simulink model "Main_bikesim_ontest2"  (R2024b)
settings: Solver=FixedStepAuto  StartTime=0.0  StopTime=inf  FixedStep=0.0005
values from neighbouring files (symbols this model uses):
  A_d = permute(A_d,[1,3,2])    [Main_sim.m]    (also in Startup_labview_v2.m; sensor_error_test_sequence.m = (eye(size(A))+Ts*A))
  Ad_t = eye(1)+Ts*A_t    [Main_sim.m]    (also in Startup_labview_v2.m = (eye(size(A_t))+Ts*A_t))
  B_d = zeros(V_n,7,1)    [Main_sim.m]    (also in Startup_labview_v2.m; sensor_error_test_sequence.m = Ts*B)
  badGPS = 0    [Main_sim.m]
  Bd_t = B_t*Ts    [Main_sim.m]    (also in Startup_labview_v2.m)
  bike_model = 1    [Main_sim.m]
  bike_params = LoadBikeParameters(bike)    [Compare_real_to_sim.m]    (also in MPC_Data_train.m = LoadBikeParameters("green"); Main_sim.m; Startup_labview_v2.m; sensor_error_test_sequence.m)
  C = mpc_outer_params.Cd    [MPC_Data_train.m]    (also in Main_sim.m = permute(C,[1,3,2]); Startup_labview_v2.m = permute(C,[1,3,2]); fromIMU2trajectory.m = (W_roll * W_roll.') / max(1, size(W_roll,2)); sensor_data_check.m = (W_roll * W_roll.') / max(1, size(W_roll,2)))
  C_t = zeros(V_n,1)    [Main_sim.m]    (also in Startup_labview_v2.m)
  counter = zeros(V_n,1)    [Main_sim.m]    (also in Startup_labview_v2.m; sensor_error_test_sequence.m = 9)
  D = mpc_outer_params.Dd    [MPC_Data_train.m]    (also in Main_sim.m = zeros(V_n,7,1); Startup_labview_v2.m = zeros(V_n,7,1))
  D_t = zeros(V_n,1)    [Main_sim.m]    (also in Startup_labview_v2.m)
  e1_max = abs(-k2*e2_max/k1)    [Startup_labview_v2.m]
  friction_coefficient = 0.004    [Main_sim.m]
  gg = 9.81    [Main_sim.m]    (also in Startup_labview_v2.m)
  hor_dis = 5    [Main_sim.m]
  I_balancing_outer = 0.0    (= 0)    [Main_sim.m]    (also in Startup_labview_v2.m; sensor_error_test_sequence.m)
  indoor = 0    [Main_sim.m]
  initial_state_estimate = initial_state    [Main_sim.m]    (also in sensor_error_test_sequence.m)
  interpolation = 0    [Main_sim.m]
  k1 = K(1)    [Startup_labview_v2.m]
  k2 = K(2)    [Startup_labview_v2.m]
  K_GPS = permute(K_GPS,[1,3,2])    [Main_sim.m]    (also in Startup_labview_v2.m)
  K_noGPS = permute(K_noGPS,[1,3,2])    [Main_sim.m]    (also in Startup_labview_v2.m)
  lambda = bike_params.lambda    [MPC_Data_train.m]    (also in sensor_error_test_sequence.m = bike_params.lambda_mod)
  lf = bike_params.lf    [MPC_Data_train.m]    (also in sensor_error_test_sequence.m = bike_params.lf_mod)
  linearizedMatrices = [Ad_t, Bd_t, C_t, D_t, V']    [Main_sim.m]
  lr = bike_params.lr    [MPC_Data_train.m]    (also in sensor_error_test_sequence.m = bike_params.lr_mod)
  P_balancing_inner = 3.5    [Main_sim.m]    (also in Startup_labview_v2.m; sensor_error_test_sequence.m)
  P_balancing_outer = 3.75    [Main_sim.m]    (also in Startup_labview_v2.m; sensor_error_test_sequence.m)
  psiref = zeros(length(Xref), 1)    [Refgeneration_test.m]
  ref_dis = 1    [Main_sim.m]    (also in differenttest.m = 0.8; differenttest_Simon.m = 0.1)
  T = [ 1,  sin(phi)*tan(th),  cos(phi)*tan(th) ... (first row only)    [Copy_of_fromIMU2trajectory.m]    (also in Main_sim.m = TransMatrix(bike_params); fromIMU2trajectory.m; sensor_error_test_sequence.m = Rz*Ry*Rx; shorttrajectory.m = table(Xref, Yref, Psiref, Vref, t, 'VariableNames', {'Xref',)
  t_ref = equal_distances / speed    [differenttest.m]    (also in differenttest_Simon.m = linspace(0, (lL-1)/Vref_test, lL)')
  Ts = 0.01    [Main_sim.m]    (also in Startup_labview_v2.m; sensor_error_test_sequence.m)
  V = round(V,1)    [Main_sim.m]    (also in Startup_labview_v2.m)
  v_init = Vref(1)    [Main_sim.m]    (also in Startup_labview_v2.m)
  Vref = zeros(length(Xref), 1)    [Refgeneration_test.m]    (also in differenttest.m = Vref_test * ones(N_line, 1); differenttest_Simon.m = Vref_test * ones(N_line, 1))
  vv = 2.6    [Main_sim.m]    (also in Refgeneration.m = table_ref.v)
  Xref = [Xref;Xref2]    [ReferenceGenerator.m]    (also in concatenate.m; differenttest.m = Xref(:); differenttest_Simon.m = interp1(s, x_path, s_eq, 'linear')')
  Yref = [Yref;Yref2]    [ReferenceGenerator.m]    (also in concatenate.m; differenttest.m = Yref(:); differenttest_Simon.m = interp1(s, y_path, s_eq, 'linear')')
undefined symbols (not defined in the file or in its folder): initial_state, pert_deltadot_state, pert_deltadot_state_fun, pert_phidot_state, pert_phidot_state_fun
libraries: simulink x11, slpidlib x4, matrix_library x1, eeGeneralControl x1
(part 1 of 2)
settings Model: PauseTimes=0.16  Creator=Hadi Hajieghrary  LastModifiedBy=oskar
settings SolverCC: MaxConsecutiveMinStep=10  ZeroCrossAlgorithm=Adaptive  AlgebraicLoopSolver=TrustRegion  AutoInsertRateTranBlk=on
settings OptimizationCC: ReuseModelBlockBuffer=off
settings DebuggingCC: AlgebraicLoopMsg=none  UnconnectedInputMsg=warning  UnconnectedOutputMsg=warning  UnconnectedLineMsg=warning
settings ModelReferenceCC: EnableRefExpFcnMdlSchedulingChecks=on
settings RTWCC: GenCodeOnly=on  GPUComputeCapability=3.5  DLArmComputeVersion=19.05

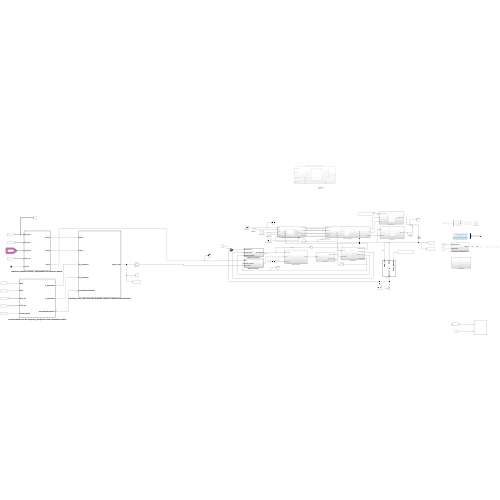
[thumbnail: Simulink's stored preview of the top-level diagram]
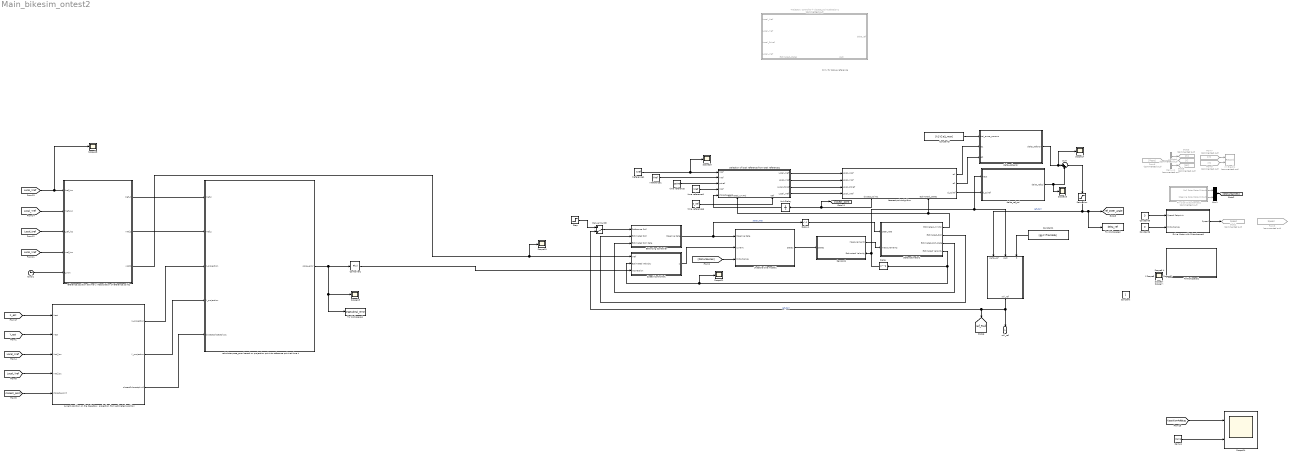
== system Main_bikesim_ontest2 ==
  note: Only for debug reference
  "  " : MATLAB Function  TreatAsAtomicUnit=on
  Balancing Controller : Subsystem  TreatAsAtomicUnit=on  SystemSampleTime=Ts
      settings: MinAlgLoopOccurrences=on
  Clock1 : Clock
  Constant1 : Constant  Value=[gg lr lf lambda]
  Constant3 : Constant  Value=[k1 k2 e1_max]  VectorParams1D=off
  Constant5 : Constant  Value=3
  Constant6 : Constant  Value=0
  Controller1 : slpidlib/PID Controller  Controller=P  Form=Parallel  TimeDomain=Discrete-time  UseExternalTs=off  SampleTime=Ts  IntegratorMethod=Forward Euler  FilterMethod=Forward Euler  ControllerParametersSource=internal  P=1  I=0  UseKiTs=off  D=0  UseExternalDerivativeSource=off  N=100  UseFilter=off  TunerSelectOption=Transfer Function Based (PID Tuner App)  InitialConditionSource=internal  InitialConditionForIntegrator=0  InitialConditionForFilter=0  DifferentiatorICPrevScaledInput=0  ExternalReset=none  TrackingMode=off  Kt=1  LimitOutput=off  SatLimitsSource=internal  UpperSaturationLimit=inf  LowerSaturationLimit=-inf  LinearizeAsGain=on  AntiWindupMode=none  Kb=1  LimitIntegrator=off  UpperIntegratorSaturationLimit=inf  LowerIntegratorSaturationLimit=-inf  POutMin=[]  POutMax=[]  IOutMin=[]  IOutMax=[]  DOutMin=[]  DOutMax=[]  NOutMin=[]  NOutMax=[]  SumOutMin=[]  SumOutMax=[]  SaturationOutMin=[]  SaturationOutMax=[]  PParamMin=[]  PParamMax=[]  IParamMin=[]  IParamMax=[]  DParamMin=[]  DParamMax=[]  NParamMin=[]  NParamMax=[]  KbParamMin=[]  KbParamMax=[]  KtParamMin=[]  KtParamMax=[]  KbOutMin=[]  KbOutMax=[]  KtOutMin=[]  KtOutMax=[]  IntegratorOutMin=[]  IntegratorOutMax=[]  FilterOutMin=[]  FilterOutMax=[]  SumI1OutMin=[]  SumI1OutMax=[]  SumI2OutMin=[]  SumI2OutMax=[]  SumI3OutMin=[]  SumI3OutMax=[]  SumI4OutMin=[]  SumI4OutMax=[]  SumDOutMin=[]  SumDOutMax=[]  DifferentiatorOutMin=[]  DifferentiatorOutMax=[]  FilterDiffOutCoefMin=[]  FilterDiffOutCoefMax=[]  ReciprocalOutMin=[]  ReciprocalOutMax=[]  SumDenOutMin=[]  SumDenOutMax=[]  SumNumOutMin=[]  SumNumOutMax=[]  DivideOutMin=[]  DivideOutMax=[]  UdiffTsProdOutMin=[]  UdiffTsProdOutMax=[]  NTsProdOutMin=[]  NTsProdOutMax=[]  UintegralTsProdOutMin=[]  UintegralTsProdOutMax=[]  UngainTsProdOutMin=[]  UngainTsProdOutMax=[]  ClampingZeroOutDataTypeStr=Inherit: Inherit via back propagation  ClampingZeroOutMin=[]  ClampingZeroOutMax=[]  FilterDenConstantOutDataTypeStr=Inherit: Inherit via back propagation  FilterDenConstantOutMin=[]  FilterDenConstantOutMax=[]  PCopyOutDataTypeStr=Inherit: Inherit via back propagation  PCopyOutMin=[]  PCopyOutMax=[]  NCopyOutDataTypeStr=Inherit: Inherit via back propagation  NCopyOutMin=[]  NCopyOutMax=[]  IntegratorContinuousStateAttributes=''  IntegratorStateMustResolveToSignalObject=off  IntegratorRTWStateStorageClass=Auto  FilterContinuousStateAttributes=''  FilterStateMustResolveToSignalObject=off  FilterRTWStateStorageClass=Auto  ParallelPVariant=InternalParameters  IdealPVariant=Disabled  IVariant=Disabled  DVariant=Disabled  IntegratorVariant=Disabled  SatVariant=Disabled  AWVariant=Disabled  PCopyVariant=Disabled  TRVariant=Disabled  FdbkBlocksVariant=Forward  IdealPFdbkVariant=Disabled  SatFdbkVariant=Disabled  DerivativeFilterVariant=Disabled  NVariant=Disabled  NCopyVariant=Disabled_SignalSpec  FilterICVariant=Disabled  IntegratorICVariant=Disabled  ExternalResetVariant=Disabled  TRSumVariant=Passthrough  SumFdbkVariant=Disabled  SumVariant=Passthrough_P  TsampFilterVariant=InternalTs  TsampNgainVariant=Passthrough  TsampIntegralVariant=Disabled_SignalSpec  ExternalSaturationOutDataTypeStr=Inherit: Same as second input  DerivativeSourceVariant=Disabled  PreIntVariant=InternalPreInt
  Delay : Delay  DelayLength=1
  Delay1 : Delay  DelayLength=1  SampleTime=Ts
  Demux1 : Demux  Commented=on  Outputs=3
  Drive Motor with Disturbance1 : Subsystem
  From3 : From  Commented=on  GotoTag=Speed  TagVisibility=global
  From5 : From  Commented=on  GotoTag=Y
  From6 : From  Commented=on  GotoTag=Pose
  From7 : From  Commented=on  GotoTag=X
  Goto1 : Goto  Commented=on  GotoTag=Speed  TagVisibility=global
  Goto3 : Goto  Commented=on  GotoTag=X
  Goto4 : Goto  Commented=on  GotoTag=Y
  Goto5 : Goto  Commented=on  GotoTag=psi
  Manual Switch : ManualSwitch  CurrentSetting=0
  Mux1 : Mux  Inputs=2
  Nearest point algrithm : Subsystem
      settings: PortSchema="{\"entries\":[{\"content\":{\"sides\":[{\"content\":{\"connectorIds\":[\"In1\",\"In2\",\"In3\",\"In4\"]},\"type\":\"ConnectorPlacement.EquallySpacedRectSide\",\"uuid\":\"e7a2fb02-f6cc-45e9-8980-79d12a8832e3\"},{\"content\":{\"connectorIds\":[\"Out1\",\"Out2\",\"Out3\"],\"side\":\"RIGHT\"},\"type\":\"ConnectorPlacement.EquallySpacedRectSide\",\"uuid\":\"304c1e91-f1f4-462f-993e-75a0bfc51b31\"},{\"content\":{\"side\":\"TOP\"},\"type\":\"ConnectorPlacement.EquallySpacedRectSide\",\"uuid\":\"75b9e2ee-7eae-4db3-b507-7ba54d105139\"},{\"content\":{\"connectorIds\":[\"Out4\",\"In5\"],\"side\":\"BOTTOM\"},\"type\":\"ConnectorPlacement.EquallySpacedRectSide\",\"uuid\":\"8b853725-4c9a-4fb3-93ea-b9b3b3cf0d57\"}]},\"type\":\"ConnectorPlacement.EquallySpacedConnector\",\"uuid\":\"c24d7268-89b5-4c3c-b432-105407319c62\"}],\"packageUris\":[\"http://schema.mathworks.com/mf0/Connector/R2020b\"],\"version\":\"1.0\"}"
  Physical Disturbances1 : Subsystem  Commented=on
  Ramp1 : simulink/Sources/Ramp  slope=2  start=0  InitialOutput=0
  Saturation : Saturate  UpperLimit=pi/4  LowerLimit=-pi/4
  Scope{,1..21} (22 alike) : Scope
  Scope24 : Scope  NumInputPorts=2
  Selection of local reference from total reference1 : Subsystem
      settings: PortSchema="{\"entries\":[{\"content\":{\"sides\":[{\"content\":{\"connectorIds\":[\"In1\",\"In2\",\"In3\",\"In4\",\"In5\"]},\"type\":\"ConnectorPlacement.EquallySpacedRectSide\",\"uuid\":\"b129a8ce-0ab0-4745-b919-7f1f6310ba72\"},{\"content\":{\"connectorIds\":[\"Out1\",\"Out2\",\"Out3\",\"Out4\"],\"side\":\"RIGHT\"},\"type\":\"ConnectorPlacement.EquallySpacedRectSide\",\"uuid\":\"29e87fb1-7c56-4cac-b724-1406f2c9c629\"},{\"content\":{\"side\":\"TOP\"},\"type\":\"ConnectorPlacement.EquallySpacedRectSide\",\"uuid\":\"7b58316d-0623-4272-bbb4-c0141a57ab8b\"},{\"content\":{\"connectorIds\":[\"In6\",\"In7\"],\"side\":\"BOTTOM\"},\"type\":\"ConnectorPlacement.EquallySpacedRectSide\",\"uuid\":\"0102ebd0-fd1a-417a-bd7a-ba724799aedf\"}]},\"type\":\"ConnectorPlacement.EquallySpacedConnector\",\"uuid\":\"fda0eb97-4558-45cb-9afe-cb94e226b238\"}],\"packageUris\":[\"http://schema.mathworks.com/mf0/Connector/R2020b\"],\"version\":\"1.0\"}"
  Sensors1 : Subsystem
      settings: PortSchema="{\"entries\":[{\"content\":{\"sides\":[{\"content\":{\"connectorIds\":[\"In1\"]},\"type\":\"ConnectorPlacement.EquallySpacedRectSide\",\"uuid\":\"0dae4ed7-efb0-46ed-930d-1e8430d36bf1\"},{\"content\":{\"connectorIds\":[\"Out1\",\"In2\"],\"side\":\"RIGHT\"},\"type\":\"ConnectorPlacement.EquallySpacedRectSide\",\"uuid\":\"ee3925d2-8342-4a47-8ecd-7ce27308bf71\"},{\"content\":{\"side\":\"TOP\"},\"type\":\"ConnectorPlacement.EquallySpacedRectSide\",\"uuid\":\"1ec196ec-b341-451c-8c31-687f560aaf31\"},{\"content\":{\"side\":\"BOTTOM\"},\"type\":\"ConnectorPlacement.EquallySpacedRectSide\",\"uuid\":\"7f3bbe3b-1797-4645-9807-b3b391e29302\"}]},\"type\":\"ConnectorPlacement.EquallySpacedConnector\",\"uuid\":\"97e5585a-d40f-4581-894d-0adc2858ded6\"}],\"packageUris\":[\"http://schema.mathworks.com/mf0/Connector/R2020b\"],\"version\":\"1.0\"}"
  Speed Controller1 : Subsystem  TreatAsAtomicUnit=on
      settings: MinAlgLoopOccurrences=on
  State estimator1 : Subsystem
  Step : Step  Time=10  After=0.15  SampleTime=0
  Sum : Sum  Inputs=|++
  To Workspace1 : ToWorkspace  VariableName=longitudinal_error  SaveFormat=Timeseries  SampleTime=-1
  To Workspace2 : ToWorkspace  VariableName=delta_ref  SaveFormat=Timeseries  SampleTime=-1
  ToWorkspace1 : Subsystem
  Trajectory controller + closest_point selection1 : Subsystem  Commented=on
      settings: PortSchema="{\"entries\":[{\"content\":{\"sides\":[{\"content\":{\"connectorIds\":[\"In1\",\"In2\",\"In3\",\"In4\"]},\"type\":\"ConnectorPlacement.EquallySpacedRectSide\",\"uuid\":\"4e12ce37-1515-428d-8e72-ea3bf7cb0ff9\"},{\"content\":{\"connectorIds\":[\"Out1\"],\"side\":\"RIGHT\"},\"type\":\"ConnectorPlacement.EquallySpacedRectSide\",\"uuid\":\"a9718efd-1612-4f51-92cf-6f7a8bfe2bda\"},{\"content\":{\"side\":\"TOP\"},\"type\":\"ConnectorPlacement.EquallySpacedRectSide\",\"uuid\":\"2b79877e-8290-4d72-b67b-1728e8961ce6\"},{\"content\":{\"connectorIds\":[\"In5\",\"In6\"],\"side\":\"BOTTOM\"},\"type\":\"ConnectorPlacement.EquallySpacedRectSide\",\"uuid\":\"2cd29579-a861-4f37-a88d-667717891393\"}]},\"type\":\"ConnectorPlacement.EquallySpacedConnector\",\"uuid\":\"1636a1cb-255f-43a6-9614-48f01e829aec\"}],\"packageUris\":[\"http://schema.mathworks.com/mf0/Connector/R2020b\"],\"version\":\"1.0\"}"
  Unit Delay : UnitDelay  SampleTime=-1  HasFrameUpgradeWarning=on
  Unstable bike model1 : Subsystem
  XY Graph1 : Record  Commented=on  FileSettingsInternal="{\"entries\":[{\"content\":{\"excelSettings\":{\"content\":{},\"type\":\"Streamout.ExcelSettings\"}},\"type\":\"Streamout.FileSettingStorage\",\"uuid\":\"\"}],\"packageUris\":[\"http:\\/\\/schema.mathworks.com\\/mf0\\/streamout_blocks\\/R2020a\"],\"version\":\"1.0\"}"  Layout=[1 1]  SignalsInternal="{\"entries\":[{\"content\":{},\"type\":\"RecordBlkView.InputSignals\",\"uuid\":\"\"}],\"packageUris\":[\"http:\\/\\/schema.mathworks.com\\/mf0\\/streamout_blocks\\/R2020a\"],\"version\":\"1.0\"}"  VisualizationBindings="{\"xyplotplugin\":{\"info\":[{\"series\":[],\"subplotID\":1}]}}"  CompatibilityTag=XY
  Xreference1 : Constant  Value=Xref
  Yreference1 : Constant  Value=Yref
  calculate pose_error based on projection point to reference point at time t : MATLAB Function  TreatAsAtomicUnit=on
  "current position on the trajectory, projection from estimated position" : MATLAB Function  TreatAsAtomicUnit=on
  delta_ref_error : Subsystem
  delta_ref_psi : Subsystem
  "reference position at time t, interpolation of reference points " : MATLAB Function  TreatAsAtomicUnit=on
  time reference : Constant  Value=psiref
  time reference1 : Constant  Value=Vref
  time reference6 : Constant  Value=t_ref
  roll_ref : Outport
  Constant : Constant  IOType=siggen
  tag scope: closest_point=global, ref_Roll=global, ref_steer_angle=global
  wires:
  State estimator1/1(Estimated_X/Y/Psi) -> Selection of local reference from total reference1/6(Estimated_X/Y/Psi), Nearest point algrithm/5(Estimated_states)
  Delay1/1 -> State estimator1/1(steer_rate)
  Unstable bike model1/1(States) -> Sensors1/1(States)
  Demux1/1 -> Goto3/1
  Balancing Controller/1(Steering Rate) -> Delay1/1, Unstable bike model1/1(Steering Rate)  "steer_rate"
  From5/1 -> XY Graph1/2
  [Disturbances] -> Unstable bike model1/3(Disturbance)
  State estimator1/2(Estimated_Roll) -> Balancing Controller/2(Estimated Roll)
  Demux1/3 -> Goto5/1
  Physical Disturbances1/2(Steering Rate State Disturb) -> Mux1/2
  Demux1/2 -> Goto4/1
  Drive Motor with Disturbance1/1(Speed) -> Goto1/1
  Mux1/1 -> [Disturbances]
  Constant5/1 -> Drive Motor with Disturbance1/1(Speed Setpoint)
  Physical Disturbances1/1(Roll Rate State Disturb) -> Mux1/1
  From7/1 -> XY Graph1/1
  Constant6/1 -> Drive Motor with Disturbance1/2(Disturbance)
  From6/1 -> Demux1/1
  State estimator1/3(Estimated_Roll_Rate) -> Balancing Controller/3(Estimated Roll Rate)
  Manual Switch/1 -> Balancing Controller/1(Reference Roll)
  Sensors1/1(Measurements) -> State estimator1/2(measurements)
  State estimator1/4(Estimated Velocity) -> Speed Controller1/2(Estimated Velocity), Scope21/1, Delay/1
  Delay/1 -> delta_ref_psi/1(Vest), "  "/2(Vest), Sensors1/2(Estimated Velocity)
  Unit Delay/1 -> Selection of local reference from total reference1/5(closest_point)
  Saturation/1 -> "  "/1(delta_ref), To Workspace2/1, [ref_steer_angle]  "ref_Roll"
  Constant1/1 -> "  "/3(bike_params)
  "  "/1(roll_ref) -> roll_ref/1, Manual Switch/2, [ref_Roll]  "ref_Roll"
  Xreference1/1 -> Scope20/1, Selection of local reference from total reference1/1(Xref)
  Yreference1/1 -> Selection of local reference from total reference1/2(Yref)
  Selection of local reference from total reference1/1(Local_Xref) -> Nearest point algrithm/1(Local_Xref)
  Selection of local reference from total reference1/2(Local_Yref) -> Nearest point algrithm/2(Local_Yref)
  Selection of local reference from total reference1/3(Local_Psiref) -> Nearest point algrithm/3(Local_Psiref)
  Nearest point algrithm/4(closest_point1) -> [closest_point], Unit Delay/1
  Constant3/1 -> delta_ref_error/1(traj_erroe_params)
  delta_ref_error/1(delta_referror) -> Scope17/1, Sum/1
  Nearest point algrithm/3(d_psiref) -> delta_ref_psi/2(d_psiref)
  delta_ref_psi/1(delta_refpsi) -> Scope16/1, Sum/2
  [X_est] -> "current position on the trajectory, projection from estimated position"/1(Xest)
  [Y_est] -> "current position on the trajectory, projection from estimated position"/2(Yest)
  "reference position at time t, interpolation of reference points "/1(Xref_t) -> calculate pose_error based on projection point to reference point at time t/1(Xref_t)
  "reference position at time t, interpolation of reference points "/2(Yref_t) -> calculate pose_error based on projection point to reference point at time t/2(Yref_t)
  "current position on the trajectory, projection from estimated position"/1(X_projection) -> calculate pose_error based on projection point to reference point at time t/3(X_projection)
  "current position on the trajectory, projection from estimated position"/2(Y_projection) -> calculate pose_error based on projection point to reference point at time t/4(Y_projection)
  "current position on the trajectory, projection from estimated position"/3(closest2closestplus1) -> calculate pose_error based on projection point to reference point at time t/5(closest2closestplus1)
  calculate pose_error based on projection point to reference point at time t/1(pose_error) -> To Workspace1/1, Scope15/1, Controller1/1
  Clock1/1 -> "reference position at time t, interpolation of reference points "/5(t_now)
  time reference/1 -> Selection of local reference from total reference1/3(psiref)
  time reference1/1 -> Selection of local reference from total reference1/4(Vref)
  [Local_Xref] -> "current position on the trajectory, projection from estimated position"/3(Xref_loc)
  [Local_Yref] -> "current position on the trajectory, projection from estimated position"/4(Yref_loc)
  [closest_point] -> "current position on the trajectory, projection from estimated position"/5(closest_point)
  Speed Controller1/1(" ") -> Unstable bike model1/2(current)
  [Xposition4debug] -> Scope24/1
  Ramp1/1 -> Scope24/2
  Selection of local reference from total reference1/4(Local_Vref) -> Nearest point algrithm/4(Local_Vref)
  time reference6/1 -> Selection of local reference from total reference1/7(tref)
  [Local_Xref] -> Scope18/1, "reference position at time t, interpolation of reference points "/1(Xref_loc)
  [Local_Yref] -> "reference position at time t, interpolation of reference points "/2(Yref_loc)
  [Local_Vref] -> "reference position at time t, interpolation of reference points "/4(vref_loc)
  [Local_tref] -> "reference position at time t, interpolation of reference points "/3(t_ref_loc)
  Sum/1 -> Saturation/1
  Nearest point algrithm/1(e1) -> delta_ref_error/2(e1)
  Nearest point algrithm/2(e2) -> delta_ref_error/3(e2)
  Controller1/1 -> Speed Controller1/3(Vcorrection)
  Step/1 -> Manual Switch/1
  "reference position at time t, interpolation of reference points "/3(vref_t) -> Speed Controller1/1(Vref), Scope19/1

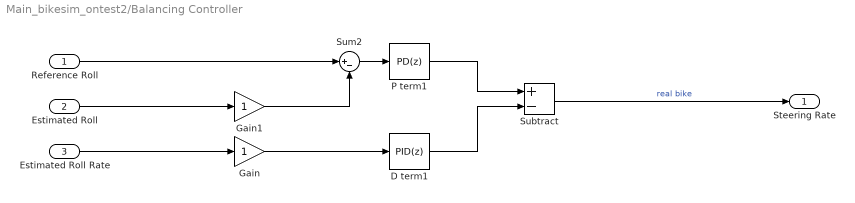
== system Main_bikesim_ontest2/Balancing Controller ==
  Reference Roll : Inport
  Estimated Roll : Inport  Port=2
  Estimated Roll Rate : Inport  Port=3
  D term1 : slpidlib/PID Controller  Controller=PID  Form=Parallel  TimeDomain=Discrete-time  UseExternalTs=off  SampleTime=Ts  IntegratorMethod=Forward Euler  FilterMethod=Forward Euler  ControllerParametersSource=internal  P=P_balancing_inner  I=0  UseKiTs=off  D=0  UseExternalDerivativeSource=off  N=100  UseFilter=off  TunerSelectOption=Transfer Function Based (PID Tuner App)  InitialConditionSource=internal  InitialConditionForIntegrator=0  InitialConditionForFilter=0  DifferentiatorICPrevScaledInput=0  ExternalReset=none  TrackingMode=off  Kt=1  LimitOutput=off  SatLimitsSource=internal  UpperSaturationLimit=inf  LowerSaturationLimit=-inf  LinearizeAsGain=on  AntiWindupMode=none  Kb=1  LimitIntegrator=off  UpperIntegratorSaturationLimit=inf  LowerIntegratorSaturationLimit=-inf  POutMin=[]  POutMax=[]  IOutMin=[]  IOutMax=[]  DOutMin=[]  DOutMax=[]  NOutMin=[]  NOutMax=[]  SumOutMin=[]  SumOutMax=[]  SaturationOutMin=[]  SaturationOutMax=[]  PParamMin=[]  PParamMax=[]  IParamMin=[]  IParamMax=[]  DParamMin=[]  DParamMax=[]  NParamMin=[]  NParamMax=[]  KbParamMin=[]  KbParamMax=[]  KtParamMin=[]  KtParamMax=[]  KbOutMin=[]  KbOutMax=[]  KtOutMin=[]  KtOutMax=[]  IntegratorOutMin=[]  IntegratorOutMax=[]  FilterOutMin=[]  FilterOutMax=[]  SumI1OutMin=[]  SumI1OutMax=[]  SumI2OutMin=[]  SumI2OutMax=[]  SumI3OutMin=[]  SumI3OutMax=[]  SumI4OutMin=[]  SumI4OutMax=[]  SumDOutMin=[]  SumDOutMax=[]  DifferentiatorOutMin=[]  DifferentiatorOutMax=[]  FilterDiffOutCoefMin=[]  FilterDiffOutCoefMax=[]  ReciprocalOutMin=[]  ReciprocalOutMax=[]  SumDenOutMin=[]  SumDenOutMax=[]  SumNumOutMin=[]  SumNumOutMax=[]  DivideOutMin=[]  DivideOutMax=[]  UdiffTsProdOutMin=[]  UdiffTsProdOutMax=[]  NTsProdOutMin=[]  NTsProdOutMax=[]  UintegralTsProdOutMin=[]  UintegralTsProdOutMax=[]  UngainTsProdOutMin=[]  UngainTsProdOutMax=[]  ClampingZeroOutDataTypeStr=Inherit: Inherit via back propagation  ClampingZeroOutMin=[]  ClampingZeroOutMax=[]  FilterDenConstantOutDataTypeStr=Inherit: Inherit via back propagation  FilterDenConstantOutMin=[]  FilterDenConstantOutMax=[]  PCopyOutDataTypeStr=Inherit: Inherit via back propagation  PCopyOutMin=[]  PCopyOutMax=[]  NCopyOutDataTypeStr=Inherit: Inherit via back propagation  NCopyOutMin=[]  NCopyOutMax=[]  IntegratorContinuousStateAttributes=''  IntegratorStateMustResolveToSignalObject=off  IntegratorRTWStateStorageClass=Auto  FilterContinuousStateAttributes=''  FilterStateMustResolveToSignalObject=off  FilterRTWStateStorageClass=Auto  ParallelPVariant=InternalParameters  IdealPVariant=Disabled  IVariant=InternalParameters  DVariant=InternalParameters  IntegratorVariant=Discrete  SatVariant=Disabled  AWVariant=Passthrough  PCopyVariant=Disabled  TRVariant=Disabled  FdbkBlocksVariant=Forward  IdealPFdbkVariant=Disabled  SatFdbkVariant=Disabled  DerivativeFilterVariant=Differentiator  NVariant=Passthrough  NCopyVariant=Disabled_SignalSpec  FilterICVariant=InternalICsDifferentiator  IntegratorICVariant=InternalICs  ExternalResetVariant=Disabled  TRSumVariant=Passthrough  SumFdbkVariant=Disabled  SumVariant=Sum_PID  TsampFilterVariant=InternalTs  TsampNgainVariant=Passthrough  TsampIntegralVariant=Disabled_SignalSpec  ExternalSaturationOutDataTypeStr=Inherit: Same as second input  DerivativeSourceVariant=ErrorSignal  PreIntVariant=InternalPreInt
  Gain : Gain
  Gain1 : Gain
  P term1 : slpidlib/PID Controller  Controller=PD  Form=Parallel  TimeDomain=Discrete-time  UseExternalTs=off  SampleTime=Ts  IntegratorMethod=Forward Euler  FilterMethod=Forward Euler  ControllerParametersSource=internal  P=P_balancing_outer  I=I_balancing_outer  UseKiTs=off  D=0  UseExternalDerivativeSource=off  N=100  UseFilter=off  TunerSelectOption=Transfer Function Based (PID Tuner App)  InitialConditionSource=internal  InitialConditionForIntegrator=0  InitialConditionForFilter=0  DifferentiatorICPrevScaledInput=0  ExternalReset=none  TrackingMode=off  Kt=1  LimitOutput=off  SatLimitsSource=internal  UpperSaturationLimit=inf  LowerSaturationLimit=-inf  LinearizeAsGain=on  AntiWindupMode=none  Kb=1  LimitIntegrator=off  UpperIntegratorSaturationLimit=inf  LowerIntegratorSaturationLimit=-inf  POutMin=[]  POutMax=[]  IOutMin=[]  IOutMax=[]  DOutMin=[]  DOutMax=[]  NOutMin=[]  NOutMax=[]  SumOutMin=[]  SumOutMax=[]  SaturationOutMin=[]  SaturationOutMax=[]  PParamMin=[]  PParamMax=[]  IParamMin=[]  IParamMax=[]  DParamMin=[]  DParamMax=[]  NParamMin=[]  NParamMax=[]  KbParamMin=[]  KbParamMax=[]  KtParamMin=[]  KtParamMax=[]  KbOutMin=[]  KbOutMax=[]  KtOutMin=[]  KtOutMax=[]  IntegratorOutMin=[]  IntegratorOutMax=[]  FilterOutMin=[]  FilterOutMax=[]  SumI1OutMin=[]  SumI1OutMax=[]  SumI2OutMin=[]  SumI2OutMax=[]  SumI3OutMin=[]  SumI3OutMax=[]  SumI4OutMin=[]  SumI4OutMax=[]  SumDOutMin=[]  SumDOutMax=[]  DifferentiatorOutMin=[]  DifferentiatorOutMax=[]  FilterDiffOutCoefMin=[]  FilterDiffOutCoefMax=[]  ReciprocalOutMin=[]  ReciprocalOutMax=[]  SumDenOutMin=[]  SumDenOutMax=[]  SumNumOutMin=[]  SumNumOutMax=[]  DivideOutMin=[]  DivideOutMax=[]  UdiffTsProdOutMin=[]  UdiffTsProdOutMax=[]  NTsProdOutMin=[]  NTsProdOutMax=[]  UintegralTsProdOutMin=[]  UintegralTsProdOutMax=[]  UngainTsProdOutMin=[]  UngainTsProdOutMax=[]  ClampingZeroOutDataTypeStr=Inherit: Inherit via back propagation  ClampingZeroOutMin=[]  ClampingZeroOutMax=[]  FilterDenConstantOutDataTypeStr=Inherit: Inherit via back propagation  FilterDenConstantOutMin=[]  FilterDenConstantOutMax=[]  PCopyOutDataTypeStr=Inherit: Inherit via back propagation  PCopyOutMin=[]  PCopyOutMax=[]  NCopyOutDataTypeStr=Inherit: Inherit via back propagation  NCopyOutMin=[]  NCopyOutMax=[]  IntegratorContinuousStateAttributes=''  IntegratorStateMustResolveToSignalObject=off  IntegratorRTWStateStorageClass=Auto  FilterContinuousStateAttributes=''  FilterStateMustResolveToSignalObject=off  FilterRTWStateStorageClass=Auto  ParallelPVariant=InternalParameters  IdealPVariant=Disabled  IVariant=Disabled  DVariant=InternalParameters  IntegratorVariant=Disabled  SatVariant=Disabled  AWVariant=Disabled  PCopyVariant=Disabled  TRVariant=Disabled  FdbkBlocksVariant=Forward  IdealPFdbkVariant=Disabled  SatFdbkVariant=Disabled  DerivativeFilterVariant=Differentiator  NVariant=Passthrough  NCopyVariant=Disabled_SignalSpec  FilterICVariant=InternalICsDifferentiator  IntegratorICVariant=Disabled  ExternalResetVariant=Disabled  TRSumVariant=Passthrough  SumFdbkVariant=Disabled  SumVariant=Sum_PD  TsampFilterVariant=InternalTs  TsampNgainVariant=Passthrough  TsampIntegralVariant=Disabled_SignalSpec  ExternalSaturationOutDataTypeStr=Inherit: Same as second input  DerivativeSourceVariant=ErrorSignal  PreIntVariant=InternalPreInt
  Subtract : Sum  Inputs=+-
  Sum2 : Sum  Inputs=|+-
  Steering Rate : Outport
  wires:
  Sum2/1 -> P term1/1
  D term1/1 -> Subtract/2
  P term1/1 -> Subtract/1
  Estimated Roll Rate/1 -> Gain/1
  Subtract/1 -> Steering Rate/1  "real bike"
  Estimated Roll/1 -> Gain1/1
  Reference Roll/1 -> Sum2/1
  Gain/1 -> D term1/1
  Gain1/1 -> Sum2/2

== system Main_bikesim_ontest2/Drive Motor with Disturbance1 ==
  Speed Setpoint : Inport
  Disturbance : Inport  Port=2
  Sum2 : Sum  Inputs=++|
  Transfer Fcn : TransferFcn  Denominator=[2 1]
  Speed : Outport
  wires:
  Sum2/1 -> Speed/1
  Transfer Fcn/1 -> Sum2/2
  Speed Setpoint/1 -> Transfer Fcn/1
  Disturbance/1 -> Sum2/1

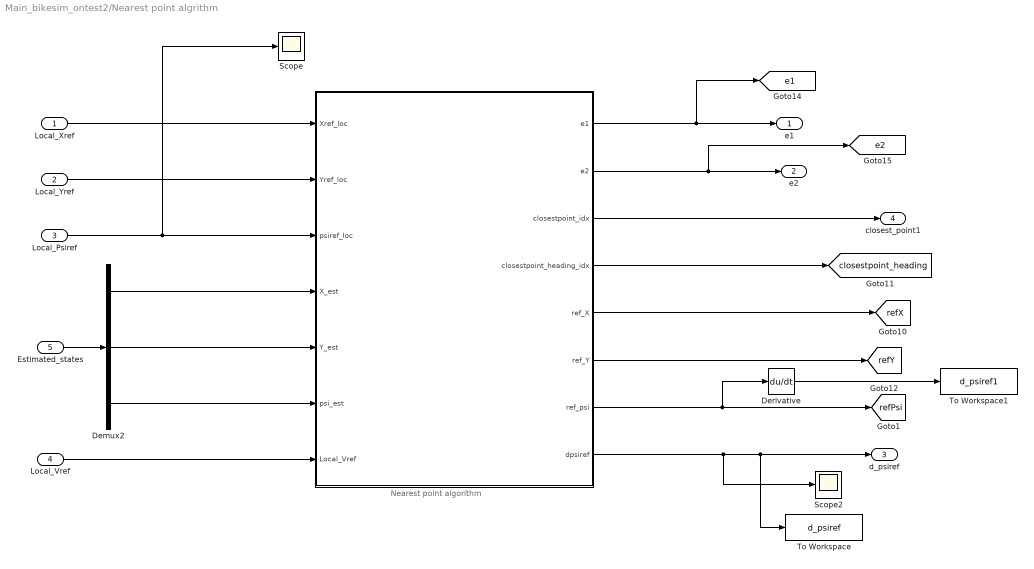
== system Main_bikesim_ontest2/Nearest point algrithm ==
  note: Nearest point algorithm
  Local_Xref : Inport
  Local_Yref : Inport  Port=2
  Local_Psiref : Inport  Port=3
  Local_Vref : Inport  Port=4
  Estimated_states : Inport  Port=5
  "  " : MATLAB Function  TreatAsAtomicUnit=on
  Demux2 : Demux  Outputs=3
  Derivative : Derivative
  Scope : Scope
  Scope2 : Scope
  To Workspace : ToWorkspace  VariableName=d_psiref  SaveFormat=Timeseries  SampleTime=-1
  To Workspace1 : ToWorkspace  VariableName=d_psiref1  SaveFormat=Timeseries  SampleTime=-1
  e1 : Outport
  e2 : Outport  Port=2
  d_psiref : Outport  Port=3
  closest_point1 : Outport  Port=4
  tag scope: closestpoint_heading=global, e1=global, e2=global, refPsi=global, refX=global, refY=global
  wires:
  "  "/7(ref_psi) -> [refPsi], Derivative/1
  "  "/5(ref_X) -> [refX]
  Demux2/1 -> "  "/4(X_est)
  Local_Yref/1 -> "  "/2(Yref_loc)
  Demux2/2 -> "  "/5(Y_est)
  "  "/6(ref_Y) -> [refY]
  Local_Psiref/1 -> Scope/1, "  "/3(psiref_loc)
  Local_Xref/1 -> "  "/1(Xref_loc)
  Estimated_states/1 -> Demux2/1
  "  "/4(closestpoint_heading_idx) -> [closestpoint_heading]
  "  "/3(closestpoint_idx) -> closest_point1/1
  "  "/8(dpsiref) -> Scope2/1, To Workspace/1, d_psiref/1
  "  "/1(e1) -> [e1], e1/1
  "  "/2(e2) -> [e2], e2/1
  Demux2/3 -> "  "/6(psi_est)
  Local_Vref/1 -> "  "/7(Local_Vref)
  Derivative/1 -> To Workspace1/1

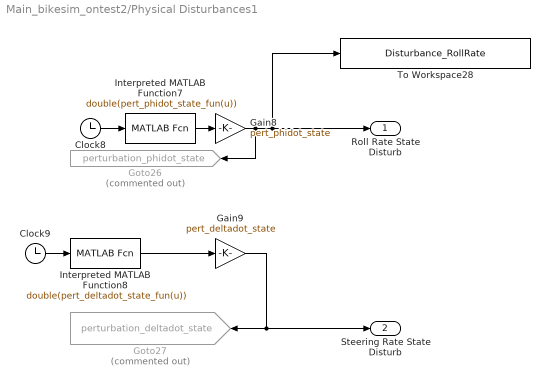
== system Main_bikesim_ontest2/Physical Disturbances1 ==
  Clock8 : Clock
  Clock9 : Clock
  Gain8 : Gain  Gain=pert_phidot_state
  Gain9 : Gain  Gain=pert_deltadot_state
  Goto26 : Goto  Commented=on  GotoTag=perturbation_phidot_state  TagVisibility=global
  Goto27 : Goto  Commented=on  GotoTag=perturbation_deltadot_state  TagVisibility=global
  Interpreted MATLAB Function7 : MATLABFcn  MATLABFcn=double(pert_phidot_state_fun(u))
  Interpreted MATLAB Function8 : MATLABFcn  MATLABFcn=double(pert_deltadot_state_fun(u))
  To Workspace28 : ToWorkspace  VariableName=Disturbance_RollRate  SaveFormat=Timeseries  SampleTime=-1
  Roll Rate State Disturb : Outport
  Steering Rate State Disturb : Outport  Port=2
  wires:
  Interpreted MATLAB Function7/1 -> Gain8/1
  Clock8/1 -> Interpreted MATLAB Function7/1
  Gain8/1 -> Goto26/1, Roll Rate State Disturb/1, To Workspace28/1
  Interpreted MATLAB Function8/1 -> Gain9/1
  Clock9/1 -> Interpreted MATLAB Function8/1
  Gain9/1 -> Steering Rate State Disturb/1, Goto27/1

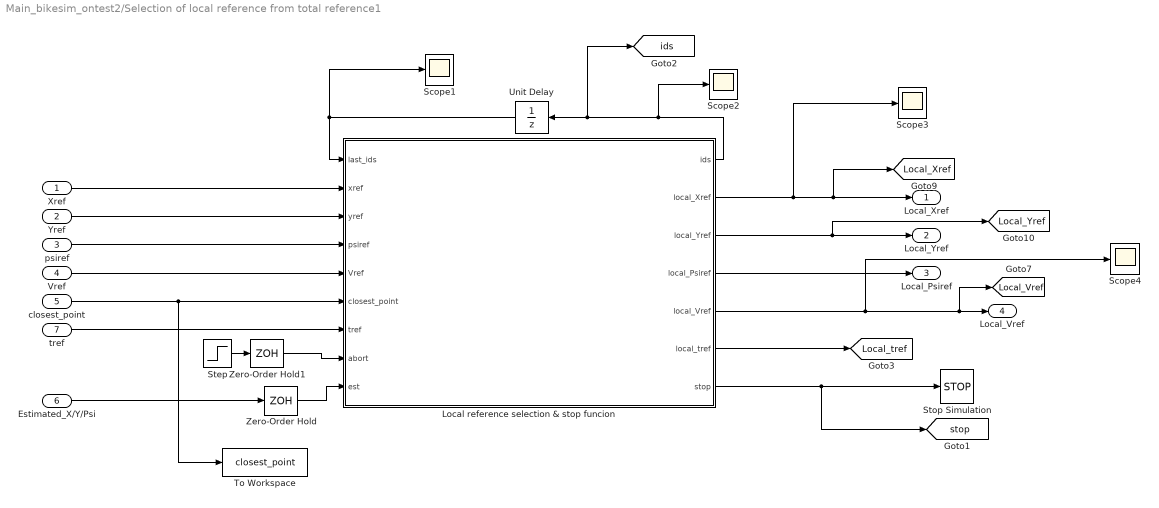
== system Main_bikesim_ontest2/Selection of local reference from total reference1 ==
  Xref : Inport
  Yref : Inport  Port=2
  psiref : Inport  Port=3
  Vref : Inport  Port=4
  closest_point : Inport  Port=5
  Estimated_X/Y/Psi : Inport  Port=6
  tref : Inport  Port=7
  Local reference selection & stop funcion : MATLAB Function  TreatAsAtomicUnit=on
  Scope{1..4} (4 alike) : Scope
  Step : Step  Time=20  After=0  SampleTime=0
  Stop Simulation : Stop
  To Workspace : ToWorkspace  VariableName=closest_point  SaveFormat=Timeseries  SampleTime=-1
  Unit Delay : UnitDelay  InitialCondition=1  SampleTime=Ts  HasFrameUpgradeWarning=on
  Zero-Order Hold : ZeroOrderHold  SampleTime=-1
  Zero-Order Hold1 : ZeroOrderHold  SampleTime=-1
  Local_Xref : Outport
  Local_Yref : Outport  Port=2
  Local_Psiref : Outport  Port=3
  Local_Vref : Outport  Port=4
  tag scope: Local_Vref=global, Local_Xref=global, Local_Yref=global, Local_tref=global, ids=global, stop=global
  wires:
  Local reference selection & stop funcion/1(ids) -> Scope2/1, [ids], Unit Delay/1
  closest_point/1 -> To Workspace/1, Local reference selection & stop funcion/6(closest_point)
  Xref/1 -> Local reference selection & stop funcion/2(xref)
  Yref/1 -> Local reference selection & stop funcion/3(yref)
  psiref/1 -> Local reference selection & stop funcion/4(psiref)
  Local reference selection & stop funcion/2(local_Xref) -> Scope3/1, Local_Xref/1, [Local_Xref]
  Local reference selection & stop funcion/3(local_Yref) -> Local_Yref/1, [Local_Yref]
  Local reference selection & stop funcion/4(local_Psiref) -> Local_Psiref/1
  Estimated_X/Y/Psi/1 -> Zero-Order Hold/1
  Zero-Order Hold/1 -> Local reference selection & stop funcion/9(est)
  Zero-Order Hold1/1 -> Local reference selection & stop funcion/8(abort)
  Step/1 -> Zero-Order Hold1/1
  Vref/1 -> Local reference selection & stop funcion/5(Vref)
  Local reference selection & stop funcion/5(local_Vref) -> Scope4/1, [Local_Vref], Local_Vref/1
  Unit Delay/1 -> Scope1/1, Local reference selection & stop funcion/1(last_ids)
  Local reference selection & stop funcion/7(stop) -> Stop Simulation/1, [stop]
  tref/1 -> Local reference selection & stop funcion/7(tref)
  Local reference selection & stop funcion/6(local_tref) -> [Local_tref]

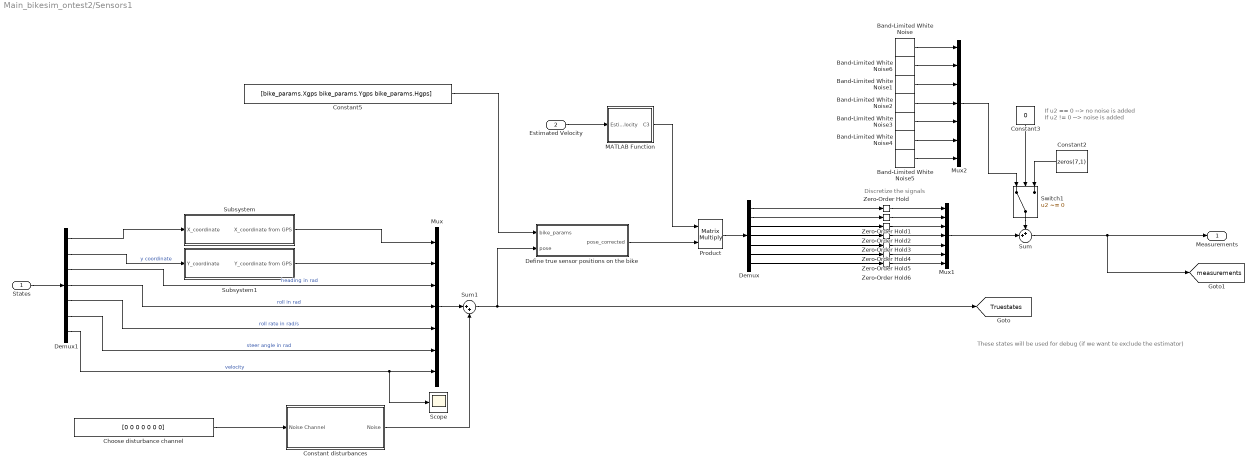
== system Main_bikesim_ontest2/Sensors1 ==
  note: These states will be used for debug (if we want te exclude the estimator)
  note: Discretize the signals
  note: If u2 == 0 --> no noise is added
      | If u2 != 0 --> noise is added
  States : Inport
  Estimated Velocity : Inport  Port=2
  Band-Limited White Noise : simulink/Sources/Band-Limited White Noise  Cov=0.001  Ts=Ts  seed=[23341]
  Band-Limited White Noise{1..6} (6 alike) : simulink/Sources/Band-Limited White Noise  Cov=0  Ts=Ts  seed=[23341]
  Choose disturbance channel : Constant  Value=[0 0 0 0 0 0 0]  VectorParams1D=off
  Constant disturbances : Subsystem
  Constant2 : Constant  Value=zeros(7,1)
  Constant3 : Constant  Value=0
  Constant5 : Constant  Value=[bike_params.Xgps bike_params.Ygps bike_params.Hgps]  VectorParams1D=off
  Define true sensor positions on the bike : MATLAB Function  TreatAsAtomicUnit=on
  Demux : Demux  Outputs=7
  Demux1 : Demux  Outputs=7
  MATLAB Function : MATLAB Function  TreatAsAtomicUnit=on
  Mux : Mux  Inputs=7
  Mux1 : Mux  Inputs=7
  Mux2 : Mux  Inputs=7
  Product : Product  Multiplication=Matrix(*)
  Scope : Scope
  Subsystem : Subsystem
  Subsystem1 : Subsystem
  Sum : Sum  Inputs=++|
  Sum1 : Sum  Inputs=|++
  Switch1 : Switch  Criteria=u2 ~= 0  SaturateOnIntegerOverflow=off  InputSameDT=off
  Zero-Order Hold : ZeroOrderHold  SampleTime=10*Ts
  Zero-Order Hold1 : ZeroOrderHold  SampleTime=10*Ts
  Zero-Order Hold{2..6} (5 alike) : ZeroOrderHold  SampleTime=Ts
  Measurements : Outport
  tag scope: Truestates=global, measurements=global
  wires:
  Sum1/1 -> [Truestates], Define true sensor positions on the bike/2(pose)
  Switch1/1 -> Sum/1
  Constant2/1 -> Switch1/3
  Constant3/1 -> Switch1/2
  Mux1/1 -> Sum/2
  Product/1 -> Demux/1
  Demux/2 -> Zero-Order Hold1/1
  Demux/4 -> Zero-Order Hold3/1
  Demux/5 -> Zero-Order Hold4/1
  Demux/6 -> Zero-Order Hold5/1
  Demux/7 -> Zero-Order Hold6/1
  Zero-Order Hold/1 -> Mux1/1
  Zero-Order Hold1/1 -> Mux1/2
  Zero-Order Hold2/1 -> Mux1/3
  Zero-Order Hold3/1 -> Mux1/4
  Zero-Order Hold4/1 -> Mux1/5
  Zero-Order Hold5/1 -> Mux1/6
  Zero-Order Hold6/1 -> Mux1/7
  Sum/1 -> [measurements], Measurements/1
  Demux/1 -> Zero-Order Hold/1
  Define true sensor positions on the bike/1(pose_corrected) -> Product/2
  Constant5/1 -> Define true sensor positions on the bike/1(bike_params)
  States/1 -> Demux1/1
  Demux1/7 -> Scope/1, Mux/7  "velocity"
  Demux1/1 -> Subsystem/1(X_coordinate)
  Demux1/5 -> Mux/5  "roll rate in rad/s"
  Demux1/4 -> Mux/4  "roll in rad"
  Demux1/3 -> Mux/3  "heading in rad"
  Demux1/6 -> Mux/6  "steer angle in rad"
  Mux2/1 -> Switch1/1
  Band-Limited White Noise/1 -> Mux2/1
  Band-Limited White Noise5/1 -> Mux2/7
  Band-Limited White Noise4/1 -> Mux2/6
  Band-Limited White Noise3/1 -> Mux2/5
  Band-Limited White Noise2/1 -> Mux2/4
  Band-Limited White Noise1/1 -> Mux2/3
  Band-Limited White Noise6/1 -> Mux2/2
  Demux/3 -> Zero-Order Hold2/1
  Mux/1 -> Sum1/1
  Choose disturbance channel/1 -> Constant disturbances/1(Noise Channel)
  Constant disturbances/1(Noise) -> Sum1/2
  Subsystem/1(X_coordinate from GPS) -> Mux/1
  Demux1/2 -> Subsystem1/1(Y_coordinate)  "y coordinate"
  Subsystem1/1(Y_coordinate from GPS) -> Mux/2
  Estimated Velocity/1 -> MATLAB Function/1(Estimated_Velocity)
  MATLAB Function/1(C3) -> Product/1

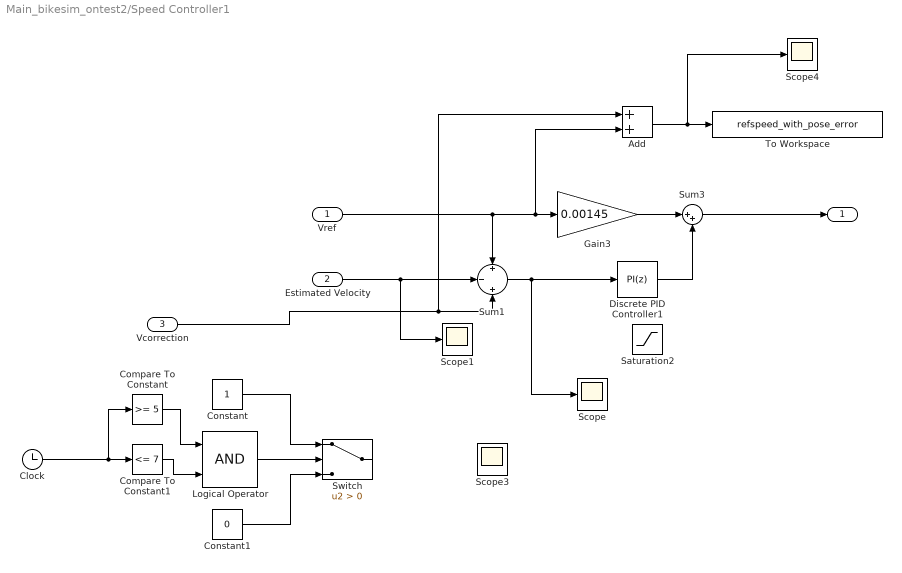
== system Main_bikesim_ontest2/Speed Controller1 ==
  Vref : Inport
  Estimated Velocity : Inport  Port=2
  Vcorrection : Inport  Port=3
  Add : Sum
  Clock : Clock
  Compare To Constant : simulink/Logic and Bit Operations/Compare To Constant  relop=>=  const=5  OutDataTypeStr=boolean
  Compare To Constant1 : simulink/Logic and Bit Operations/Compare To Constant  relop=<=  const=7  OutDataTypeStr=boolean
  Constant : Constant
  Constant1 : Constant  Value=0
  Discrete PID Controller1 : slpidlib/PID Controller  Controller=PI  Form=Parallel  TimeDomain=Discrete-time  UseExternalTs=off  SampleTime=Ts  IntegratorMethod=Forward Euler  FilterMethod=Forward Euler  ControllerParametersSource=internal  P=2  I=0.5  UseKiTs=off  D=0  UseExternalDerivativeSource=off  N=100  UseFilter=on  TunerSelectOption=Transfer Function Based (PID Tuner App)  InitialConditionSource=internal  InitialConditionForIntegrator=0  InitialConditionForFilter=0  DifferentiatorICPrevScaledInput=0  ExternalReset=none  TrackingMode=off  Kt=1  LimitOutput=off  SatLimitsSource=internal  UpperSaturationLimit=inf  LowerSaturationLimit=-inf  LinearizeAsGain=off  AntiWindupMode=none  Kb=1  LimitIntegrator=off  UpperIntegratorSaturationLimit=inf  LowerIntegratorSaturationLimit=-inf  POutMin=[]  POutMax=[]  IOutMin=[]  IOutMax=[]  DOutMin=[]  DOutMax=[]  NOutMin=[]  NOutMax=[]  SumOutMin=[]  SumOutMax=[]  SaturationOutMin=[]  SaturationOutMax=[]  PParamMin=[]  PParamMax=[]  IParamMin=[]  IParamMax=[]  DParamMin=[]  DParamMax=[]  NParamMin=[]  NParamMax=[]  KbParamMin=[]  KbParamMax=[]  KtParamMin=[]  KtParamMax=[]  KbOutMin=[]  KbOutMax=[]  KtOutMin=[]  KtOutMax=[]  IntegratorOutMin=[]  IntegratorOutMax=[]  FilterOutMin=[]  FilterOutMax=[]  SumI1OutMin=[]  SumI1OutMax=[]  SumI2OutMin=[]  SumI2OutMax=[]  SumI3OutMin=[]  SumI3OutMax=[]  SumI4OutMin=[]  SumI4OutMax=[]  SumDOutMin=[]  SumDOutMax=[]  DifferentiatorOutMin=[]  DifferentiatorOutMax=[]  FilterDiffOutCoefMin=[]  FilterDiffOutCoefMax=[]  ReciprocalOutMin=[]  ReciprocalOutMax=[]  SumDenOutMin=[]  SumDenOutMax=[]  SumNumOutMin=[]  SumNumOutMax=[]  DivideOutMin=[]  DivideOutMax=[]  UdiffTsProdOutMin=[]  UdiffTsProdOutMax=[]  NTsProdOutMin=[]  NTsProdOutMax=[]  UintegralTsProdOutMin=[]  UintegralTsProdOutMax=[]  UngainTsProdOutMin=[]  UngainTsProdOutMax=[]  ClampingZeroOutDataTypeStr=Inherit: Inherit via back propagation  ClampingZeroOutMin=[]  ClampingZeroOutMax=[]  FilterDenConstantOutDataTypeStr=Inherit: Inherit via back propagation  FilterDenConstantOutMin=[]  FilterDenConstantOutMax=[]  PCopyOutDataTypeStr=Inherit: Inherit via back propagation  PCopyOutMin=[]  PCopyOutMax=[]  NCopyOutDataTypeStr=Inherit: Inherit via back propagation  NCopyOutMin=[]  NCopyOutMax=[]  IntegratorContinuousStateAttributes=''  IntegratorStateMustResolveToSignalObject=off  IntegratorRTWStateStorageClass=Auto  FilterContinuousStateAttributes=''  FilterStateMustResolveToSignalObject=off  FilterRTWStateStorageClass=Auto  ParallelPVariant=InternalParameters  IdealPVariant=Disabled  IVariant=InternalParameters  DVariant=Disabled  IntegratorVariant=Discrete  SatVariant=Disabled  AWVariant=Passthrough  PCopyVariant=Disabled  TRVariant=Disabled  FdbkBlocksVariant=Forward  IdealPFdbkVariant=Disabled  SatFdbkVariant=Disabled  DerivativeFilterVariant=Disabled  NVariant=Disabled  NCopyVariant=Disabled_SignalSpec  FilterICVariant=Disabled  IntegratorICVariant=InternalICs  ExternalResetVariant=Disabled  TRSumVariant=Passthrough  SumFdbkVariant=Disabled  SumVariant=Sum_PI  TsampFilterVariant=InternalTs  TsampNgainVariant=Passthrough  TsampIntegralVariant=Disabled_SignalSpec  ExternalSaturationOutDataTypeStr=Inherit: Same as second input  DerivativeSourceVariant=Disabled  PreIntVariant=InternalPreInt
  Gain3 : Gain  Gain=0.00145
  Logical Operator : Logic  AllPortsSameDT=off  OutDataTypeStr=boolean
  Saturation2 : Saturate  UpperLimit=4  LowerLimit=0
  Scope{,1,3..4} (4 alike) : Scope
  Sum1 : Sum  Inputs=+|-|+
  Sum3 : Sum  Inputs=|++
  Switch : Switch  Criteria=u2 > Threshold  SaturateOnIntegerOverflow=off  InputSameDT=off
  To Workspace : ToWorkspace  VariableName=refspeed_with_pose_error  SaveFormat=Timeseries  SampleTime=-1
  " " : Outport
  wires:
  Estimated Velocity/1 -> Scope1/1, Sum1/2
  Discrete PID Controller1/1 -> Sum3/2
  Sum3/1 -> " "/1
  Vref/1 -> Add/2, Gain3/1, Sum1/1
  Gain3/1 -> Sum3/1
  Clock/1 -> Compare To Constant/1, Compare To Constant1/1
  Compare To Constant/1 -> Logical Operator/1
  Compare To Constant1/1 -> Logical Operator/2
  Logical Operator/1 -> Switch/2
  Constant/1 -> Switch/1
  Constant1/1 -> Switch/3
  Add/1 -> Scope4/1, To Workspace/1
  Sum1/1 -> Discrete PID Controller1/1, Scope/1
  Vcorrection/1 -> Add/1, Sum1/3

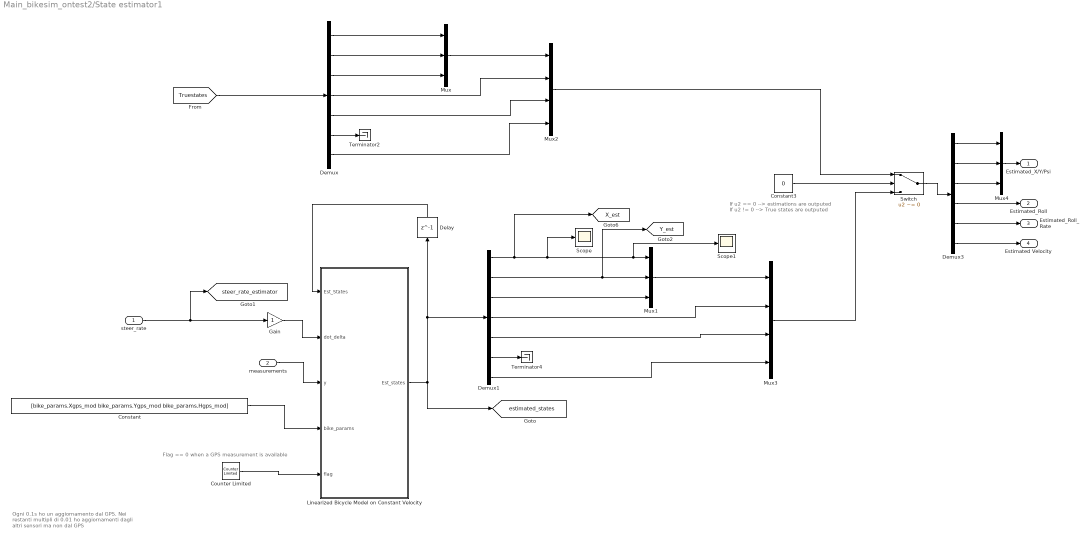
== system Main_bikesim_ontest2/State estimator1 ==
  note: Ogni 0.1s ho un aggiornamento dal GPS. Nei restanti multipli di 0.01 ho aggiornamenti dagli altri sensori ma non dal GPS
  note: Flag == 0 when a GPS measurement is available
  note: If u2 == 0 --> estimations are outputed
      | If u2 != 0 --> True states are outputed
  steer_rate : Inport
  measurements : Inport  Port=2
  Constant : Constant  Value=[bike_params.Xgps_mod bike_params.Ygps_mod bike_params.Hgps_mod]  VectorParams1D=off
  Constant3 : Constant  Value=0
  Counter Limited : simulink/Sources/Counter Limited  uplimit=counter  tsamp=Ts
  Delay : Delay  DelayLength=1  InitialCondition=[initial_state_estimate.x initial_state_estimate.y initial_state_estimate.heading initial_state.roll initial_state.roll_rate initial_state.steering v_init]  SampleTime=Ts
  Demux : Demux  Outputs=7
  Demux1 : Demux  Outputs=7
  Demux3 : Demux  Outputs=6
  Gain : Gain
  Linearized Bicycle Model on Constant Velocity : MATLAB Function  TreatAsAtomicUnit=on
  Mux : Mux  Inputs=3
  Mux1 : Mux  Inputs=3
  Mux2 : Mux
  Mux3 : Mux
  Mux4 : Mux  Inputs=3
  Scope : Scope
  Scope1 : Scope
  Switch : Switch  Criteria=u2 ~= 0  SaturateOnIntegerOverflow=off  InputSameDT=off
  Terminator2 : Terminator
  Terminator4 : Terminator
  Estimated_X/Y/Psi : Outport  VectorParamsAs1DForOutWhenUnconnected=off
  Estimated_Roll : Outport  Port=2  VectorParamsAs1DForOutWhenUnconnected=off
  Estimated_Roll_Rate : Outport  Port=3  VectorParamsAs1DForOutWhenUnconnected=off
  Estimated Velocity : Outport  Port=4  VectorParamsAs1DForOutWhenUnconnected=off
  tag scope: X_est=global, Y_est=global, estimated_states=global, steer_rate_estimator=global
  wires:
  Demux/3 -> Mux/3
  Gain/1 -> Linearized Bicycle Model on Constant Velocity/2(dot_delta)
  Demux1/5 -> Mux3/3
  Delay/1 -> Linearized Bicycle Model on Constant Velocity/1(Est_States)
  steer_rate/1 -> [steer_rate_estimator], Gain/1
  Demux1/2 -> [Y_est], Mux1/2
  Demux/1 -> Mux/1
  Demux1/1 -> [X_est], Scope/1, Scope1/1, Mux1/1
  Demux/2 -> Mux/2
  Demux1/7 -> Mux3/4
  Demux/7 -> Mux2/4
  Demux/6 -> Terminator2/1
  Mux/1 -> Mux2/1
  Mux2/1 -> Switch/1
  Mux3/1 -> Switch/3
  Constant3/1 -> Switch/2
  Demux/4 -> Mux2/2
  Demux/5 -> Mux2/3
  Mux1/1 -> Mux3/1
  Demux1/4 -> Mux3/2
  Switch/1 -> Demux3/1
  Demux3/1 -> Mux4/1
  Demux3/2 -> Mux4/2
  Demux3/3 -> Mux4/3
  Mux4/1 -> Estimated_X/Y/Psi/1
  Demux3/4 -> Estimated_Roll/1
  Demux3/5 -> Estimated_Roll_Rate/1
  Counter Limited/1 -> Linearized Bicycle Model on Constant Velocity/5(flag)
  Demux1/3 -> Mux1/3
  Constant/1 -> Linearized Bicycle Model on Constant Velocity/4(bike_params)
  measurements/1 -> Linearized Bicycle Model on Constant Velocity/3(y)
  [Truestates] -> Demux/1
  Linearized Bicycle Model on Constant Velocity/1(Est_states) -> Delay/1, Demux1/1, [estimated_states]
  Demux1/6 -> Terminator4/1
  Demux3/6 -> Estimated Velocity/1

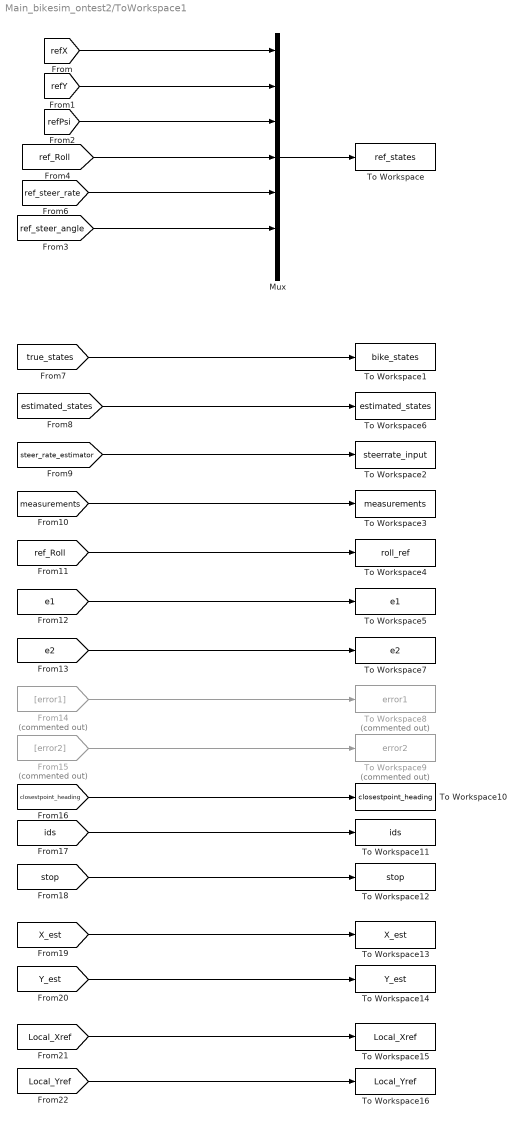
== system Main_bikesim_ontest2/ToWorkspace1 ==
  From14 : From  Commented=on  GotoTag=error1
  From15 : From  Commented=on  GotoTag=error2
  Mux : Mux  Inputs=7
  To Workspace : ToWorkspace  VariableName=ref_states  SaveFormat=Timeseries  SampleTime=-1
  To Workspace1 : ToWorkspace  VariableName=bike_states  SaveFormat=Timeseries  SampleTime=-1
  To Workspace10 : ToWorkspace  VariableName=closestpoint_heading  SaveFormat=Timeseries  SampleTime=-1
  To Workspace11 : ToWorkspace  VariableName=ids  SaveFormat=Timeseries  SampleTime=-1
  To Workspace12 : ToWorkspace  VariableName=stop  SaveFormat=Timeseries  SampleTime=-1
  To Workspace13 : ToWorkspace  VariableName=X_est  SaveFormat=Timeseries  SampleTime=-1
  To Workspace14 : ToWorkspace  VariableName=Y_est  SaveFormat=Timeseries  SampleTime=-1
  To Workspace15 : ToWorkspace  VariableName=Local_Xref  SaveFormat=Timeseries  SampleTime=-1
  To Workspace16 : ToWorkspace  VariableName=Local_Yref  SaveFormat=Timeseries  SampleTime=-1
  To Workspace2 : ToWorkspace  VariableName=steerrate_input  SaveFormat=Timeseries  SampleTime=-1
  To Workspace3 : ToWorkspace  VariableName=measurements  SaveFormat=Timeseries  SampleTime=-1
  To Workspace4 : ToWorkspace  VariableName=roll_ref  SaveFormat=Timeseries  SampleTime=-1
  To Workspace5 : ToWorkspace  VariableName=e1  SaveFormat=Timeseries  SampleTime=-1
  To Workspace6 : ToWorkspace  VariableName=estimated_states  SaveFormat=Timeseries  SampleTime=-1
  To Workspace7 : ToWorkspace  VariableName=e2  SaveFormat=Timeseries  SampleTime=-1
  To Workspace8 : ToWorkspace  Commented=on  VariableName=error1  SaveFormat=Timeseries  SampleTime=-1
  To Workspace9 : ToWorkspace  Commented=on  VariableName=error2  SaveFormat=Timeseries  SampleTime=-1
  wires:
  [refX] -> Mux/1
  [refY] -> Mux/2
  [refPsi] -> Mux/3
  [ref_Roll] -> Mux/4
  Mux/1 -> To Workspace/1
  [true_states] -> To Workspace1/1
  [ref_steer_angle] -> Mux/6
  [ref_steer_rate] -> Mux/5
  [estimated_states] -> To Workspace6/1
  [steer_rate_estimator] -> To Workspace2/1
  [measurements] -> To Workspace3/1
  [ref_Roll] -> To Workspace4/1
  [e1] -> To Workspace5/1
  [e2] -> To Workspace7/1
  From14/1 -> To Workspace8/1
  From15/1 -> To Workspace9/1
  [closestpoint_heading] -> To Workspace10/1
  [ids] -> To Workspace11/1
  [stop] -> To Workspace12/1
  [Y_est] -> To Workspace14/1
  [X_est] -> To Workspace13/1
  [Local_Xref] -> To Workspace15/1
  [Local_Yref] -> To Workspace16/1

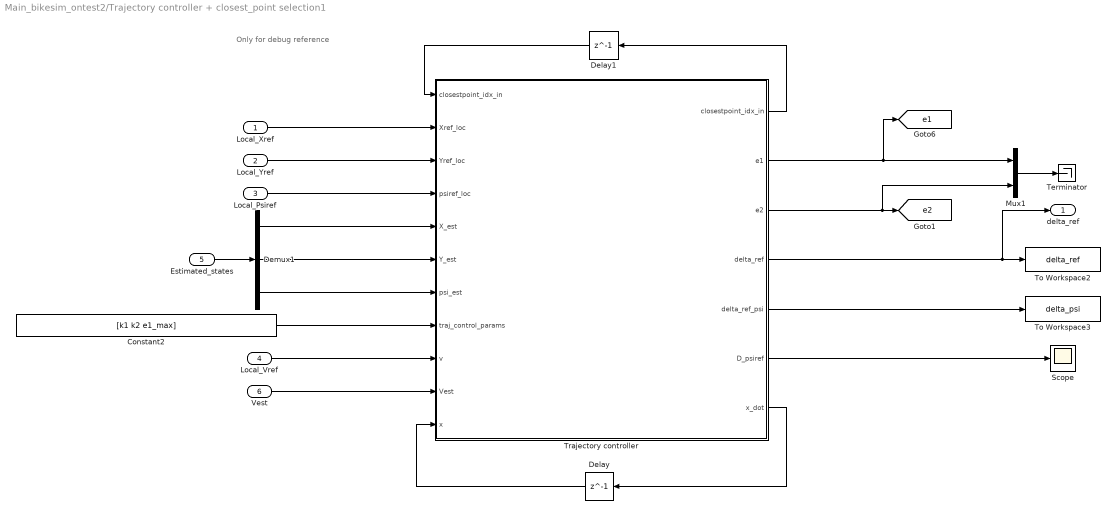
== system Main_bikesim_ontest2/Trajectory controller + closest_point selection1 ==
  note: Only for debug reference
  Local_Xref : Inport
  Local_Yref : Inport  Port=2
  Local_Psiref : Inport  Port=3
  Local_Vref : Inport  Port=4
  Estimated_states : Inport  Port=5
  Vest : Inport  Port=6
  Constant2 : Constant  Value=[k1 k2 e1_max]
  Delay : Delay  DelayLength=1  SampleTime=Ts
  Delay1 : Delay  DelayLength=1  InitialCondition=2  SampleTime=Ts
  Demux1 : Demux  Outputs=3
  Mux1 : Mux  Inputs=2
  Scope : Scope
  Terminator : Terminator
  To Workspace2 : ToWorkspace  VariableName=delta_ref  SaveFormat=Timeseries  SampleTime=-1
  To Workspace3 : ToWorkspace  VariableName=delta_psi  SaveFormat=Timeseries  SampleTime=-1
  Trajectory controller : MATLAB Function  TreatAsAtomicUnit=on
  delta_ref : Outport
  tag scope: e1=global, e2=global
  wires:
  Mux1/1 -> Terminator/1
  Trajectory controller/7(x_dot) -> Delay/1
  Constant2/1 -> Trajectory controller/8(traj_control_params)
  Estimated_states/1 -> Demux1/1
  Trajectory controller/2(e1) -> [e1], Mux1/1
  Local_Yref/1 -> Trajectory controller/3(Yref_loc)
  Local_Psiref/1 -> Trajectory controller/4(psiref_loc)
  Demux1/1 -> Trajectory controller/5(X_est)
  Demux1/2 -> Trajectory controller/6(Y_est)
  Delay/1 -> Trajectory controller/11(x)
  Local_Xref/1 -> Trajectory controller/2(Xref_loc)
  Trajectory controller/3(e2) -> Mux1/2, [e2]
  Demux1/3 -> Trajectory controller/7(psi_est)
  Trajectory controller/1(closestpoint_idx_in) -> Delay1/1
  Delay1/1 -> Trajectory controller/1("closestpoint_idx_in ")
  Trajectory controller/5(delta_ref_psi) -> To Workspace3/1
  Trajectory controller/6(D_psiref) -> Scope/1
  Trajectory controller/4(delta_ref) -> delta_ref/1, To Workspace2/1
  Vest/1 -> Trajectory controller/10(Vest)
  Local_Vref/1 -> Trajectory controller/9(v)
